simulink model "RobotModel"  (R2021b)
settings: Solver=VariableStepAuto  StartTime=0.0  StopTime=10.0  RelTol=1e-3
values from neighbouring files (symbols this model uses):
  U_alim = 24.0    [RobotModel.sldd]    (also in Robot_mdl_Workspace.m = 24)
undefined symbols (not defined in the file or in its folder): L_roue, R_roue
settings Model: DataDictionary=RobotModel.sldd  EnableAccessToBaseWorkspace=off  Creator=hugo  LastModifiedBy=hugo
settings SolverCC: AlgebraicLoopSolver=TrustRegion
settings DataIOCC: SaveOutput=off  SaveTime=off  ReturnWorkspaceOutputs=off
settings DebuggingCC: SFMachineParentedDataDiag=warning  ArithmeticOperatorsInVariantConditions=warning
settings ModelReferenceCC: ModelReferenceMinAlgLoopOccurrences=on
settings SFSimCC: SimUseLocalCustomCode=off  CustomCodeUndefinedFunction=UseInterfaceOnly
settings RTWCC: RTWUseLocalCustomCode=off

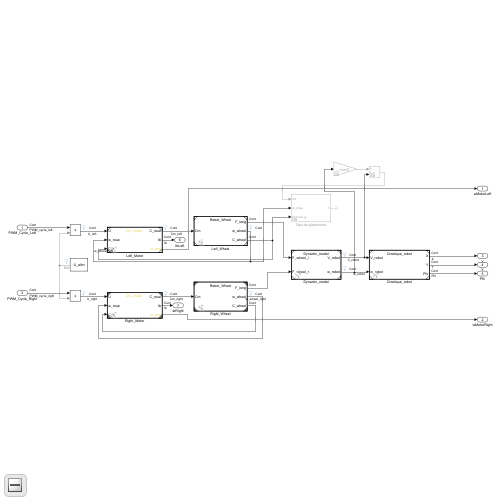
[thumbnail: Simulink's stored preview of the top-level diagram]
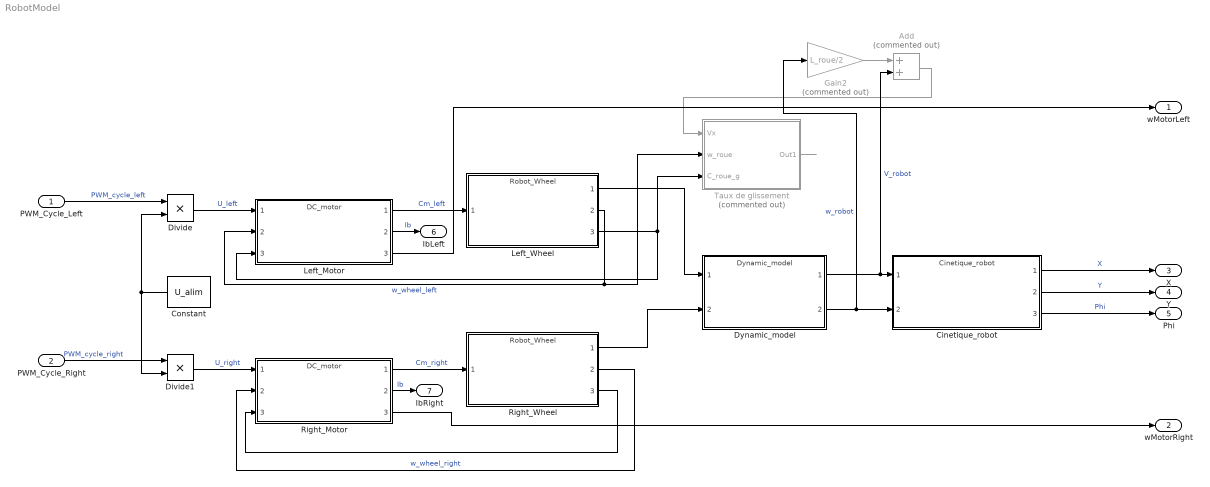
== system RobotModel ==
  PWM_Cycle_Left : Inport  OutDataTypeStr=double  PortDimensions=1  SampleTime=0
  PWM_Cycle_Right : Inport  Port=2  OutDataTypeStr=double  PortDimensions=1  SampleTime=0
  Add : Sum  Commented=on
  Cinetique_robot : ModelReference  ModelNameDialog=Cinetique_robot.slx  SimulationMode=Normal  ModelReferenceVersion=1.54
  Constant : Constant  Value=U_alim  SampleTime=0
  Divide : Product  Inputs=**
  Divide1 : Product  Inputs=**
  Dynamic_model : ModelReference  ModelNameDialog=Dynamic_model.slx  SimulationMode=Normal  ModelReferenceVersion=1.8
  Gain2 : Gain  Commented=on  Gain=L_roue/2
  Left_Motor : ModelReference  ModelNameDialog=DC_motor.slx  SimulationMode=Normal  ModelReferenceVersion=8.2
  Left_Wheel : ModelReference  ModelNameDialog=Robot_Wheel.slx  SimulationMode=Normal  ModelReferenceVersion=1.9
  Right_Motor : ModelReference  ModelNameDialog=DC_motor.slx  SimulationMode=Normal  ModelReferenceVersion=8.2
  Right_Wheel : ModelReference  ModelNameDialog=Robot_Wheel.slx  SimulationMode=Normal  ModelReferenceVersion=1.9
  Taux de glissement : Subsystem  Commented=on
  wMotorLeft : Outport  OutDataTypeStr=double  PortDimensions=1  SampleTime=0  VectorParamsAs1DForOutWhenUnconnected=off
  wMotorRight : Outport  Port=2  OutDataTypeStr=double  PortDimensions=1  SampleTime=0  VectorParamsAs1DForOutWhenUnconnected=off
  X : Outport  Port=3  OutDataTypeStr=double  PortDimensions=1  SampleTime=0  VectorParamsAs1DForOutWhenUnconnected=off
  Y : Outport  Port=4  OutDataTypeStr=double  PortDimensions=1  SampleTime=0  VectorParamsAs1DForOutWhenUnconnected=off
  Phi : Outport  Port=5  OutDataTypeStr=double  PortDimensions=1  SampleTime=0  VectorParamsAs1DForOutWhenUnconnected=off
  IbLeft : Outport  Port=6  OutDataTypeStr=double  PortDimensions=1  SampleTime=0
  IbRight : Outport  Port=7  OutDataTypeStr=double  PortDimensions=1  SampleTime=0
  wires:
  Cinetique_robot/1 -> X/1  "X"
  Left_Wheel/2 -> Taux de glissement/2(w_roue), Left_Motor/2  "w_wheel_left"
  Add/1 -> Taux de glissement/1(Vx)
  Constant/1 -> Divide/2, Divide1/2
  Dynamic_model/2 -> Cinetique_robot/2, Gain2/1  "w_robot"
  Cinetique_robot/2 -> Y/1  "Y"
  Divide/1 -> Left_Motor/1  "U_left"
  Left_Wheel/3 -> Left_Motor/3, Taux de glissement/3(C_roue_g)
  Right_Wheel/1 -> Dynamic_model/2
  Gain2/1 -> Add/1
  Cinetique_robot/3 -> Phi/1  "Phi"
  Right_Wheel/2 -> Right_Motor/2  "w_wheel_right"
  PWM_Cycle_Right/1 -> Divide1/1  "PWM_cycle_right"
  Right_Wheel/3 -> Right_Motor/3
  Dynamic_model/1 -> Cinetique_robot/1, Add/2  "V_robot"
  PWM_Cycle_Left/1 -> Divide/1  "PWM_cycle_left"
  Divide1/1 -> Right_Motor/1  "U_right"
  Left_Motor/1 -> Left_Wheel/1  "Cm_left"
  Right_Motor/1 -> Right_Wheel/1  "Cm_right"
  Left_Wheel/1 -> Dynamic_model/1
  Taux de glissement/1(Out1) -> ?
  Left_Motor/2 -> IbLeft/1  "Ib"
  Right_Motor/2 -> IbRight/1  "Ib"
  Left_Motor/3 -> wMotorLeft/1
  Right_Motor/3 -> wMotorRight/1

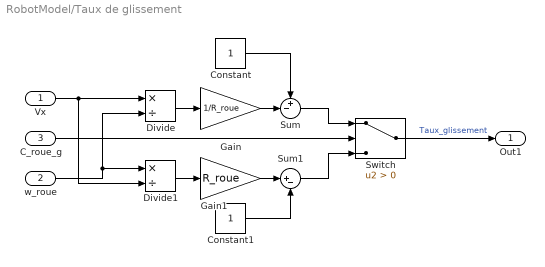
== system RobotModel/Taux de glissement ==
  Vx : Inport
  w_roue : Inport  Port=2
  C_roue_g : Inport  Port=3
  Constant : Constant
  Constant1 : Constant
  Divide : Product  Inputs=*/
  Divide1 : Product  Inputs=*/
  Gain : Gain  Gain=1/R_roue
  Gain1 : Gain  Gain=R_roue
  Sum : Sum  Inputs=+-|
  Sum1 : Sum  Inputs=|+-
  Switch : Switch  Criteria=u2 > Threshold
  Out1 : Outport  VectorParamsAs1DForOutWhenUnconnected=off
  wires:
  Sum1/1 -> Switch/3
  Constant1/1 -> Sum1/2
  Gain1/1 -> Sum1/1
  Divide1/1 -> Gain1/1
  Constant/1 -> Sum/1
  Sum/1 -> Switch/1
  Gain/1 -> Sum/2
  Divide/1 -> Gain/1
  w_roue/1 -> Divide/2, Divide1/1
  Vx/1 -> Divide/1, Divide1/2
  Switch/1 -> Out1/1  "Taux_glissement"
  C_roue_g/1 -> Switch/2
